simulink model "CoreXY_combined_feedback_model_XY"  (R2024b)
settings: Solver=VariableStepAuto  StartTime=0.0  StopTime=max(data.Time_ms_)/1000  RelTol=1e-3
undefined symbols (not defined in the file or in its folder): A_X, B_X, C_X, D_X, Kd_X, Kd_Y, Ki_X, Ki_Y, Kp_X, Kp_Y, N_X, N_Y
libraries: slpidlib x2
settings Model: Creator=trent  LastModifiedBy=mauro
settings OptimizationCC: ReuseModelBlockBuffer=off
settings DebuggingCC: UnconnectedInputMsg=warning  UnconnectedOutputMsg=warning  UnconnectedLineMsg=warning
settings ModelReferenceCC: EnableRefExpFcnMdlSchedulingChecks=on
settings RTWCC: GPUComputeCapability=3.5  DLArmComputeVersion=19.05

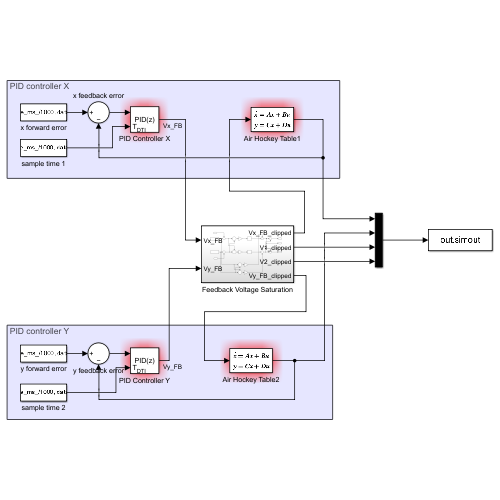
[thumbnail: Simulink's stored preview of the top-level diagram]
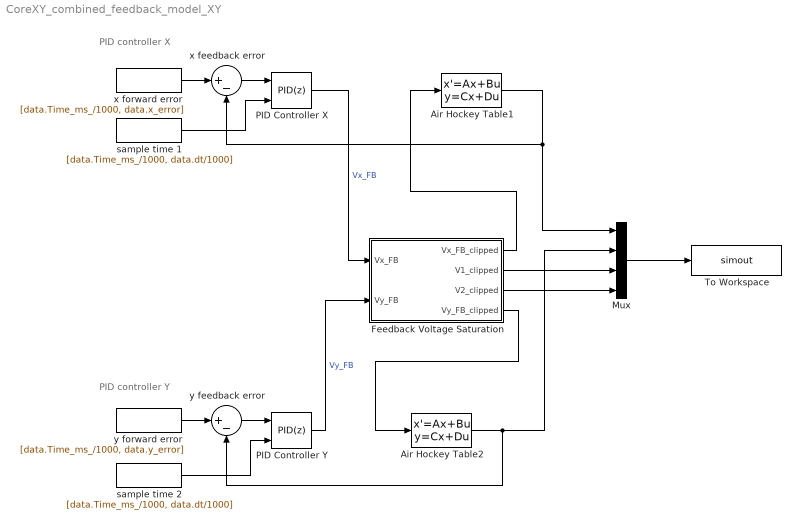
== system CoreXY_combined_feedback_model_XY ==
  note: PID controller X
  note: PID controller Y
  Air Hockey Table1 : StateSpace  A=A_X  B=B_X  C=C_X  D=D_X  InitialCondition=[0;0;0]
  Air Hockey Table2 : StateSpace  A=A_X  B=B_X  C=C_X  D=D_X  InitialCondition=[0;0;0]
  Feedback Voltage Saturation : Subsystem
  Mux : Mux
  PID Controller X : slpidlib/PID Controller  Controller=PID  Form=Parallel  TimeDomain=Discrete-time  UseExternalTs=on  SampleTime=-1  IntegratorMethod=Forward Euler  FilterMethod=Forward Euler  ControllerParametersSource=internal  P=Kp_X  I=Ki_X  UseKiTs=off  D=Kd_X  UseExternalDerivativeSource=off  N=N_X  UseFilter=on  TunerSelectOption=Transfer Function Based (PID Tuner App)  InitialConditionSource=internal  InitialConditionForIntegrator=0  InitialConditionForFilter=0  DifferentiatorICPrevScaledInput=0  ExternalReset=none  TrackingMode=off  Kt=1  LimitOutput=off  SatLimitsSource=internal  UpperSaturationLimit=inf  LowerSaturationLimit=-inf  LinearizeAsGain=on  AntiWindupMode=none  Kb=1  LimitIntegrator=off  UpperIntegratorSaturationLimit=inf  LowerIntegratorSaturationLimit=-inf  POutMin=[]  POutMax=[]  IOutMin=[]  IOutMax=[]  DOutMin=[]  DOutMax=[]  NOutMin=[]  NOutMax=[]  SumOutMin=[]  SumOutMax=[]  SaturationOutMin=[]  SaturationOutMax=[]  PParamMin=[]  PParamMax=[]  IParamMin=[]  IParamMax=[]  DParamMin=[]  DParamMax=[]  NParamMin=[]  NParamMax=[]  KbParamMin=[]  KbParamMax=[]  KtParamMin=[]  KtParamMax=[]  KbOutMin=[]  KbOutMax=[]  KtOutMin=[]  KtOutMax=[]  IntegratorOutMin=[]  IntegratorOutMax=[]  FilterOutMin=[]  FilterOutMax=[]  SumI1OutMin=[]  SumI1OutMax=[]  SumI2OutMin=[]  SumI2OutMax=[]  SumI3OutMin=[]  SumI3OutMax=[]  SumI4OutMin=[]  SumI4OutMax=[]  SumDOutMin=[]  SumDOutMax=[]  DifferentiatorOutMin=[]  DifferentiatorOutMax=[]  FilterDiffOutCoefMin=[]  FilterDiffOutCoefMax=[]  ReciprocalOutMin=[]  ReciprocalOutMax=[]  SumDenOutMin=[]  SumDenOutMax=[]  SumNumOutMin=[]  SumNumOutMax=[]  DivideOutMin=[]  DivideOutMax=[]  UdiffTsProdOutMin=[]  UdiffTsProdOutMax=[]  NTsProdOutMin=[]  NTsProdOutMax=[]  UintegralTsProdOutMin=[]  UintegralTsProdOutMax=[]  UngainTsProdOutMin=[]  UngainTsProdOutMax=[]  ClampingZeroOutDataTypeStr=Inherit: Inherit via back propagation  ClampingZeroOutMin=[]  ClampingZeroOutMax=[]  FilterDenConstantOutDataTypeStr=Inherit: Inherit via back propagation  FilterDenConstantOutMin=[]  FilterDenConstantOutMax=[]  PCopyOutDataTypeStr=Inherit: Inherit via back propagation  PCopyOutMin=[]  PCopyOutMax=[]  NCopyOutDataTypeStr=Inherit: Inherit via back propagation  NCopyOutMin=[]  NCopyOutMax=[]  IntegratorContinuousStateAttributes=''  IntegratorStateMustResolveToSignalObject=off  IntegratorRTWStateStorageClass=Auto  FilterContinuousStateAttributes=''  FilterStateMustResolveToSignalObject=off  FilterRTWStateStorageClass=Auto  ParallelPVariant=InternalParameters  IdealPVariant=Disabled  IVariant=InternalParameters  DVariant=InternalParameters  IntegratorVariant=Discrete  SatVariant=Disabled  AWVariant=Passthrough  PCopyVariant=Disabled  TRVariant=Disabled  FdbkBlocksVariant=Forward  IdealPFdbkVariant=Disabled  SatFdbkVariant=Disabled  DerivativeFilterVariant=ForwardEulerFilter  NVariant=InternalParameters  NCopyVariant=Disabled  FilterICVariant=InternalICsFilter  IntegratorICVariant=InternalICs  ExternalResetVariant=Disabled  TRSumVariant=Passthrough  SumFdbkVariant=Disabled  SumVariant=Sum_PID  TsampFilterVariant=ExternalTs  TsampNgainVariant=ExternalTs  TsampIntegralVariant=ExternalTs  ExternalSaturationOutDataTypeStr=Inherit: Same as second input  DerivativeSourceVariant=ErrorSignal  PreIntVariant=InternalPreInt
  PID Controller Y : slpidlib/PID Controller  Controller=PID  Form=Parallel  TimeDomain=Discrete-time  UseExternalTs=on  SampleTime=-1  IntegratorMethod=Forward Euler  FilterMethod=Forward Euler  ControllerParametersSource=internal  P=Kp_Y  I=Ki_Y  UseKiTs=off  D=Kd_Y  UseExternalDerivativeSource=off  N=N_Y  UseFilter=on  TunerSelectOption=Transfer Function Based (PID Tuner App)  InitialConditionSource=internal  InitialConditionForIntegrator=0  InitialConditionForFilter=0  DifferentiatorICPrevScaledInput=0  ExternalReset=none  TrackingMode=off  Kt=1  LimitOutput=off  SatLimitsSource=internal  UpperSaturationLimit=inf  LowerSaturationLimit=-inf  LinearizeAsGain=on  AntiWindupMode=none  Kb=1  LimitIntegrator=off  UpperIntegratorSaturationLimit=inf  LowerIntegratorSaturationLimit=-inf  POutMin=[]  POutMax=[]  IOutMin=[]  IOutMax=[]  DOutMin=[]  DOutMax=[]  NOutMin=[]  NOutMax=[]  SumOutMin=[]  SumOutMax=[]  SaturationOutMin=[]  SaturationOutMax=[]  PParamMin=[]  PParamMax=[]  IParamMin=[]  IParamMax=[]  DParamMin=[]  DParamMax=[]  NParamMin=[]  NParamMax=[]  KbParamMin=[]  KbParamMax=[]  KtParamMin=[]  KtParamMax=[]  KbOutMin=[]  KbOutMax=[]  KtOutMin=[]  KtOutMax=[]  IntegratorOutMin=[]  IntegratorOutMax=[]  FilterOutMin=[]  FilterOutMax=[]  SumI1OutMin=[]  SumI1OutMax=[]  SumI2OutMin=[]  SumI2OutMax=[]  SumI3OutMin=[]  SumI3OutMax=[]  SumI4OutMin=[]  SumI4OutMax=[]  SumDOutMin=[]  SumDOutMax=[]  DifferentiatorOutMin=[]  DifferentiatorOutMax=[]  FilterDiffOutCoefMin=[]  FilterDiffOutCoefMax=[]  ReciprocalOutMin=[]  ReciprocalOutMax=[]  SumDenOutMin=[]  SumDenOutMax=[]  SumNumOutMin=[]  SumNumOutMax=[]  DivideOutMin=[]  DivideOutMax=[]  UdiffTsProdOutMin=[]  UdiffTsProdOutMax=[]  NTsProdOutMin=[]  NTsProdOutMax=[]  UintegralTsProdOutMin=[]  UintegralTsProdOutMax=[]  UngainTsProdOutMin=[]  UngainTsProdOutMax=[]  ClampingZeroOutDataTypeStr=Inherit: Inherit via back propagation  ClampingZeroOutMin=[]  ClampingZeroOutMax=[]  FilterDenConstantOutDataTypeStr=Inherit: Inherit via back propagation  FilterDenConstantOutMin=[]  FilterDenConstantOutMax=[]  PCopyOutDataTypeStr=Inherit: Inherit via back propagation  PCopyOutMin=[]  PCopyOutMax=[]  NCopyOutDataTypeStr=Inherit: Inherit via back propagation  NCopyOutMin=[]  NCopyOutMax=[]  IntegratorContinuousStateAttributes=''  IntegratorStateMustResolveToSignalObject=off  IntegratorRTWStateStorageClass=Auto  FilterContinuousStateAttributes=''  FilterStateMustResolveToSignalObject=off  FilterRTWStateStorageClass=Auto  ParallelPVariant=InternalParameters  IdealPVariant=Disabled  IVariant=InternalParameters  DVariant=InternalParameters  IntegratorVariant=Discrete  SatVariant=Disabled  AWVariant=Passthrough  PCopyVariant=Disabled  TRVariant=Disabled  FdbkBlocksVariant=Forward  IdealPFdbkVariant=Disabled  SatFdbkVariant=Disabled  DerivativeFilterVariant=ForwardEulerFilter  NVariant=InternalParameters  NCopyVariant=Disabled  FilterICVariant=InternalICsFilter  IntegratorICVariant=InternalICs  ExternalResetVariant=Disabled  TRSumVariant=Passthrough  SumFdbkVariant=Disabled  SumVariant=Sum_PID  TsampFilterVariant=ExternalTs  TsampNgainVariant=ExternalTs  TsampIntegralVariant=ExternalTs  ExternalSaturationOutDataTypeStr=Inherit: Same as second input  DerivativeSourceVariant=ErrorSignal  PreIntVariant=InternalPreInt
  To Workspace : ToWorkspace  VariableName=simout  SaveFormat=Timeseries  SampleTime=-1
  sample time 1 : FromWorkspace  VariableName=[data.Time_ms_/1000, data.dt/1000]
  sample time 2 : FromWorkspace  VariableName=[data.Time_ms_/1000, data.dt/1000]
  x feedback error : Sum  Inputs=|+-
  x forward error : FromWorkspace  VariableName=[data.Time_ms_/1000, data.x_error]
  y feedback error : Sum  Inputs=|+-
  y forward error : FromWorkspace  VariableName=[data.Time_ms_/1000, data.y_error]
  wires:
  x feedback error/1 -> PID Controller X/1
  x forward error/1 -> x feedback error/1
  Feedback Voltage Saturation/1(Vx_FB_clipped) -> Air Hockey Table1/1
  Air Hockey Table1/1 -> Mux/1, x feedback error/2
  Feedback Voltage Saturation/4(Vy_FB_clipped) -> Air Hockey Table2/1
  Air Hockey Table2/1 -> Mux/2, y feedback error/2
  y forward error/1 -> y feedback error/1
  y feedback error/1 -> PID Controller Y/1
  Mux/1 -> To Workspace/1
  PID Controller Y/1 -> Feedback Voltage Saturation/2(Vy_FB)  "Vy_FB"
  PID Controller X/1 -> Feedback Voltage Saturation/1(Vx_FB)  "Vx_FB"
  Feedback Voltage Saturation/2(V1_clipped) -> Mux/3
  Feedback Voltage Saturation/3(V2_clipped) -> Mux/4
  sample time 1/1 -> PID Controller X/2
  sample time 2/1 -> PID Controller Y/2

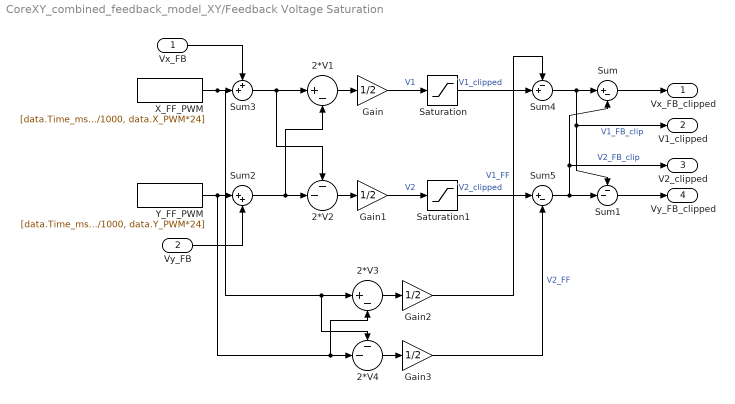
== system CoreXY_combined_feedback_model_XY/Feedback Voltage Saturation ==
  Vx_FB : Inport
  Vy_FB : Inport  Port=2
  2*V1 : Sum  Inputs=|+-
  2*V2 : Sum  Inputs=--|
  2*V3 : Sum  Inputs=|+-
  2*V4 : Sum  Inputs=--|
  Gain{,1..3} (4 alike) : Gain  Gain=1/2
  Saturation : Saturate  UpperLimit=24  LowerLimit=-24
  Saturation1 : Saturate  UpperLimit=24  LowerLimit=-24
  Sum : Sum  Inputs=|+-
  Sum1 : Sum  Inputs=--|
  Sum2 : Sum  Inputs=|++
  Sum3 : Sum  Inputs=++|
  Sum4 : Sum  Inputs=-+|
  Sum5 : Sum  Inputs=|+-
  X_FF_PWM : FromWorkspace  VariableName=[data.Time_ms_/1000, data.X_PWM*24]
  Y_FF_PWM : FromWorkspace  VariableName=[data.Time_ms_/1000, data.Y_PWM*24]
  Vx_FB_clipped : Outport
  V1_clipped : Outport  Port=2
  V2_clipped : Outport  Port=3
  Vy_FB_clipped : Outport  Port=4
  wires:
  Sum/1 -> Vx_FB_clipped/1
  Saturation1/1 -> Sum5/1  "V2_clipped"
  Sum1/1 -> Vy_FB_clipped/1
  2*V2/1 -> Gain1/1
  2*V1/1 -> Gain/1
  Gain/1 -> Saturation/1  "V1"
  Vy_FB/1 -> Sum2/2
  Saturation/1 -> Sum4/2  "V1_clipped"
  Gain1/1 -> Saturation1/1  "V2"
  Sum3/1 -> 2*V2/1, 2*V1/1
  Vx_FB/1 -> Sum3/1
  Sum2/1 -> 2*V1/2, 2*V2/2
  Sum5/1 -> V2_clipped/1, Sum/2, Sum1/2  "V2_FB_clip"
  Sum4/1 -> Sum/1, V1_clipped/1, Sum1/1  "V1_FB_clip"
  Y_FF_PWM/1 -> 2*V3/2, 2*V4/2, Sum2/1
  X_FF_PWM/1 -> 2*V4/1, 2*V3/1, Sum3/2
  2*V4/1 -> Gain3/1
  2*V3/1 -> Gain2/1
  Gain2/1 -> Sum4/1  "V1_FF"
  Gain3/1 -> Sum5/2  "V2_FF"
